simulink model "GDFLIB_FilterFIR_BAM"  (Simulink 9.3)
settings: Solver=VariableStepAuto  StartTime=0.0  StopTime=10.0  RelTol=1e-3
settings Model: Creator=nxa18952  LastModifiedBy=nxa18952
settings DataIOCC: SaveFormat=Dataset  SignalLoggingSaveFormat=Dataset  ReturnWorkspaceOutputs=on
settings OptimizationCC: LifeSpan=auto
settings DebuggingCC: UnderspecifiedInitializationDetection=Simplified  MergeDetectMultiDrivingBlocksExec=error  FcnCallInpInsideContextMsg=error  SFUnexpectedBacktrackingDiag=error  SFNoUnconditionalDefaultTransitionDiag=error  SFExecutionAtInitializationDiag=warning  ArithmeticOperatorsInVariantConditions=error
settings HardwareCC: ProdBitPerPointer=64  ProdBitPerSizeT=64  ProdBitPerPtrDiffT=64  ProdLargestAtomicFloat=Float  ProdIntDivRoundTo=Zero  ProdEndianess=LittleEndian  ProdWordSize=64  ProdHWDeviceType=Intel->x86-64 (Windows64)
settings ModelReferenceCC: PropagateSignalLabelsOutOfModel=on
settings SFSimCC: SimUseLocalCustomCode=on
settings RTWCC: RTWUseLocalCustomCode=on
settings CodeAppCC: StateflowObjectComments=off
settings GRTTargetCC: TargetLangStandard=C99 (ISO)  CombineOutputUpdateFcns=on  GRTInterface=off
settings ConfigComp: CovMetricSettings=dwe  CovHtmlReporting=off  CovSaveCumulativeToWorkspaceVar=off  CovSaveSingleToWorkspaceVar=off  CovExternalEMLEnable=on

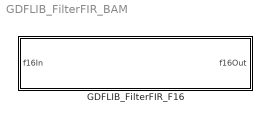
== system GDFLIB_FilterFIR_BAM ==
  GDFLIB_FilterFIR_F16 : Subsystem  TreatAsAtomicUnit=on  mask(GDFLIB_FilterFIR_F16){u16Order=3, pCoefBuf=2^15*[0.25 0.25 0.25 0.25 0]}
      mask prompts: u16Order "u16Order (FIR filter order)"; pCoefBuf "pCoefBuf (FIR filter coefficients buffer. The array stores (u16Order + 1) filter coefficients.
To use this block for code generation, add one extra element after the last filter coefficient
and make sure the array is aligned to a 32-bit boundary.)"
      mask help: Finite impulse response filter in 16-bit fixed-point fractional implementation. Refer to the AMMCLIB User's Guide for further details.
      mask init:
      | if ~evalin('base','exist(''tS8'',''var'')')
      |   if (2 ~= exist('SWLIBS_Typedefs.mat','file'))
      |       error('File SWLIBS_Typedefs.mat is not on the Matlab path. Please add the AMMCLIB "bam" folder in the Matlab Search Path.');
      |   else
      |       evalin('base', 'load(''SWLIBS_Typedefs.mat'')');
      |   end
      | end
      settings: RTWSystemCode=Inline
      mask Display: pos = get_param(gcb, 'Position');width = pos(3) - pos(1); height = pos(4) - pos(2);tX=width/2;tY=height - 8;color('black');text(tX,tY, 'GDFLIB_FilterFIR_F16', 'horizontalAlignment', 'center');

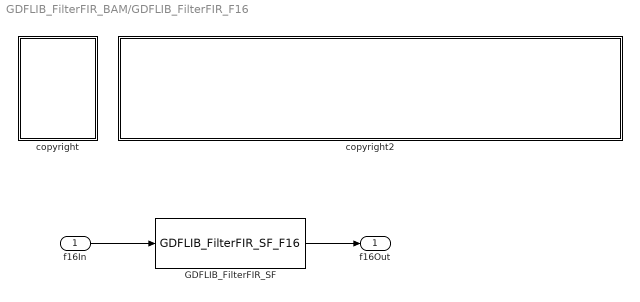
== system GDFLIB_FilterFIR_BAM/GDFLIB_FilterFIR_F16 ==
  f16In : Inport  OutDataTypeStr=int16
  GDFLIB_FilterFIR_SF : S-Function  FunctionName=GDFLIB_FilterFIR_SF_F16  Parameters=u16Order,pCoefBuf  SFunctionDeploymentMode=off  EnableBusSupport=off
  copyright : Subsystem
      mask Display: text(10,90,'FILE:');text(10,75,'DESRIPTION:');text(10,60,'COPYRIGHT:');text(10,45,'VERSION:');text(10,30,'DATE:')
  copyright2 : Subsystem
      mask Display: text(10,90,'GDFLIB_FilterFIR_BAM_F16.mdl');text(10,75,'FIR filter.');text(10,60,'NXP 2020');text(10,45,'1.0');text(10,30,'18-Mar-2020');
  f16Out : Outport
  wires:
  f16In/1 -> GDFLIB_FilterFIR_SF/1
  GDFLIB_FilterFIR_SF/1 -> f16Out/1

== system GDFLIB_FilterFIR_BAM/GDFLIB_FilterFIR_F16/copyright ==

== system GDFLIB_FilterFIR_BAM/GDFLIB_FilterFIR_F16/copyright2 ==
